simulink model "block_2ndorder_forcecont"  (R2017b)
settings: Solver=VariableStepAuto  StartTime=0.0  StopTime=1000  RelTol=1e-3
settings Model: Creator=Nick  LastModifiedBy=Nick

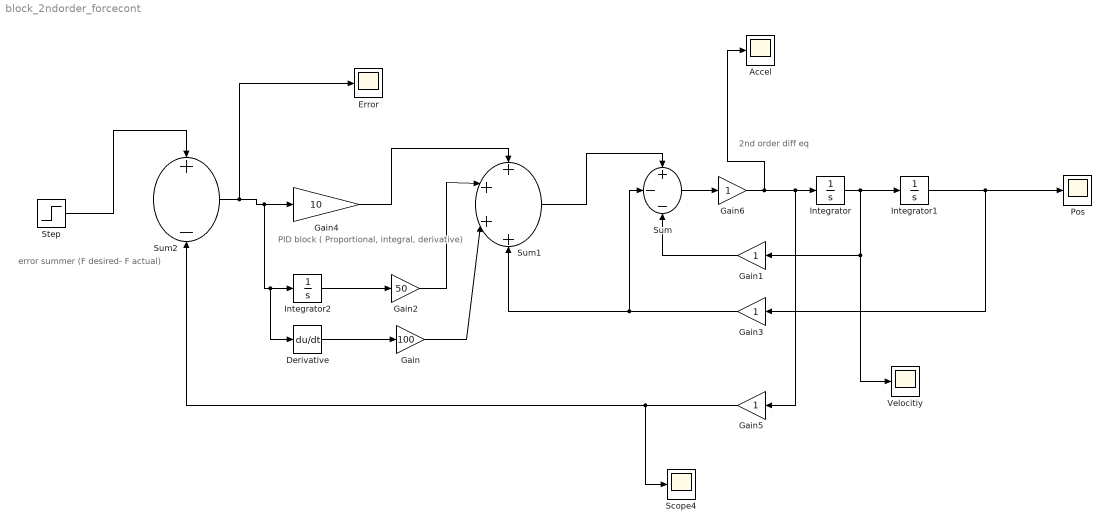
== system block_2ndorder_forcecont ==
  note: 2nd order diff eq
  note: PID block ( Proportional, integral, derivative)
  note: error summer (F desired- F actual)
  Accel : Scope
  Derivative : Derivative
  Error : Scope
  Gain : Gain  Gain=100
  Gain{1,3,5..6} (4 alike) : Gain
  Gain2 : Gain  Gain=50
  Gain4 : Gain  Gain=10
  Integrator : Integrator
  Integrator1 : Integrator
  Integrator2 : Integrator
  Pos : Scope
  Scope4 : Scope
  Step : Step  SampleTime=0
  Sum : Sum  Inputs=+--
  Sum1 : Sum  Inputs=++++
  Sum2 : Sum  Inputs=+-
  Velocitiy : Scope
  wires:
  Integrator/1 -> Gain1/1, Velocitiy/1, Integrator1/1
  Integrator1/1 -> Gain3/1, Pos/1
  Sum/1 -> Gain6/1
  Gain3/1 -> Sum1/4, Sum/2
  Gain1/1 -> Sum/3
  Integrator2/1 -> Gain2/1
  Derivative/1 -> Gain/1
  Gain4/1 -> Sum1/1
  Sum2/1 -> Error/1, Derivative/1, Integrator2/1, Gain4/1
  Gain5/1 -> Scope4/1, Sum2/2
  Gain6/1 -> Accel/1, Gain5/1, Integrator/1
  Step/1 -> Sum2/1
  Sum1/1 -> Sum/1
  Gain2/1 -> Sum1/2
  Gain/1 -> Sum1/3
